simulink library "Lib_Piccolo"  (R2018b)
settings: Solver=VariableStepAuto  StartTime=0.0  StopTime=10.0  RelTol=1e-3
values from neighbouring files (symbols this model uses):
  AccelErrInt2Brakes = 0.15    [SimulationControlConfig16P.m]    (also in SimulationControlConfig16P_F0.m; SimulationControlConfig16P_F2.m; SimulationControlConfig16P_LEGACY.m; SimulationControlConfigTAILLESS.m = 0.2)
  AileronMax = 25    [SimulationControlConfig16P.m]    (also in SimulationControlConfig16P_F0.m; SimulationControlConfig16P_F2.m; SimulationControlConfig16P_LEGACY.m; SimulationControlConfigTAILLESS.m)
  AileronPower = 0.00268    [SimulationControlConfig16P.m]    (also in SimulationControlConfig16P_F0.m; SimulationControlConfig16P_F2.m; SimulationControlConfig16P_LEGACY.m; SimulationControlConfigTAILLESS.m = 0.002266)
  AileronSurfaceMax = 45    [SimulationControlConfig16P.m]    (also in SimulationControlConfig16P_F0.m; SimulationControlConfig16P_F2.m; SimulationControlConfig16P_LEGACY.m; SimulationControlConfigTAILLESS_CGAFT_F0.m = 25)
  AileronTrim = 0    [SimulationControlConfig16P.m]    (also in SimulationControlConfig16P_F0.m; SimulationControlConfig16P_F2.m; SimulationControlConfig16P_LEGACY.m; SimulationControlConfigTAILLESS.m)
  Alt = 1000 + TerrainHeight    [SimulationStateConfig.m]
  AltCruise_m = Alt * 0.3048    [SimulationControlConfig16P.m]    (also in SimulationControlConfig16P_F2.m; SimulationControlConfigTAILLESS.m = Alt/3.28084; SimulationControlConfigTAILLESS_CGAFT_F0.m = 640; SimulationControlConfigTAILLESS_CGFWD_F0.m = 640)
  AltitudeRate2PitchCmdIntegratorInit = 0.1    [SimulationControlPre.m]
  AltMax = 10000    [SimulationControlConfig16P.m]    (also in SimulationControlConfig16P_F0.m; SimulationControlConfig16P_F2.m; SimulationControlConfig16P_LEGACY.m; SimulationControlConfigTAILLESS.m)
  AltMaxAccel = 2.5    [SimulationControlConfig16P.m]    (also in SimulationControlConfig16P_F0.m = 2; SimulationControlConfig16P_F2.m = 2; SimulationControlConfig16P_LEGACY.m = 0.9; SimulationControlConfigTAILLESS.m = 2)
  AltMin = 0    [SimulationControlConfig16P.m]    (also in SimulationControlConfig16P_F0.m; SimulationControlConfig16P_F2.m; SimulationControlConfig16P_LEGACY.m; SimulationControlConfigTAILLESS.m)
  AltRateCmd2Pitch = 0.26    [SimulationControlConfig16P.m]    (also in SimulationControlConfig16P_F0.m = 0.35; SimulationControlConfig16P_F2.m = 0.35; SimulationControlConfig16P_LEGACY.m = 0.6; SimulationControlConfigTAILLESS.m = 0.9)
  AltRateError2Pitch = 0.34    [SimulationControlConfig16P.m]    (also in SimulationControlConfig16P_F0.m = 0.61; SimulationControlConfig16P_F2.m = 0.61; SimulationControlConfig16P_LEGACY.m = 0.4; SimulationControlConfigTAILLESS.m = 0.3)
  AltRateErrorInt2Pitch = 0.61    [SimulationControlConfig16P.m]    (also in SimulationControlConfig16P_F0.m = 0.28; SimulationControlConfig16P_F2.m = 0.28; SimulationControlConfig16P_LEGACY.m = 0.45; SimulationControlConfigTAILLESS.m = 0.15)
  AltRateLpfCutOff = 3    [SimulationControlConfig16P.m]    (also in SimulationControlConfig16P_F0.m; SimulationControlConfig16P_F2.m; SimulationControlConfig16P_LEGACY.m; SimulationControlConfigTAILLESS.m = 5)
  AutoNosegear2Rudder = 26    [SimulationControlConfig16P.m]    (also in SimulationControlConfig16P_F0.m; SimulationControlConfig16P_F2.m; SimulationControlConfig16P_LEGACY.m; SimulationControlConfigTAILLESS.m = 25.2)
  b = 5.54    [SimulationControlConfig16P.m]    (also in SimulationControlConfig16P_F0.m; SimulationControlConfig16P_F2.m; SimulationControlConfig16P_LEGACY.m; SimulationControlConfigTAILLESS.m = 2.37)
  Bank2AileronIntegratorInit = 0    [SimulationControlPre.m]
  BankMax_User = BankMax_User/180*pi    (= 0.610865238198)    [SimulationControlConfig16P.m]    (also in SimulationControlConfig16P_F0.m = 0.523598775598; SimulationControlConfig16P_F2.m = 0.523598775598; SimulationControlConfig16P_LEGACY.m = 0.523598775598; SimulationControlConfigTAILLESS.m = 0.558505360638)
  baseLegFlaps = 20    [SimulationControlConfig16P.m]    (also in SimulationControlConfig16P_F0.m; SimulationControlConfig16P_F2.m = 15; SimulationControlConfig16P_LEGACY.m = 0; SimulationControlConfigTAILLESS.m = 0)
  C = GeneticOpt.C    [SimulationCostFunction.m]
  c = Sw/b    (= 0.841696750903)    [SimulationControlConfig16P.m]    (also in SimulationControlConfig16P_F0.m; SimulationControlConfig16P_F2.m; SimulationControlConfig16P_LEGACY.m; SimulationControlConfigTAILLESS.m = 0.354008438819)
  cell2WheelFactorMG = 5.98    [SimulationSensorConfig16P_LEGACY.m]
  cell2WheelFactorNG = 1    [SimulationSensorConfig16P_LEGACY.m]
  cellSatMaxMG = 15000    [SimulationSensorConfig16P.m]    (also in SimulationSensorConfig16P_LEGACY.m; SimulationSensorConfigTAILLESS7P.m; SimulationSensorConfigUTAIL7P.m)
  cellSatMaxNG = 1000    [SimulationSensorConfig16P.m]    (also in SimulationSensorConfig16P_LEGACY.m; SimulationSensorConfigTAILLESS7P.m; SimulationSensorConfigUTAIL7P.m)
  cellSatMinMG = -15000    [SimulationSensorConfig16P.m]    (also in SimulationSensorConfig16P_LEGACY.m; SimulationSensorConfigTAILLESS7P.m; SimulationSensorConfigUTAIL7P.m)
  cellSatMinNG = -1000    [SimulationSensorConfig16P.m]    (also in SimulationSensorConfig16P_LEGACY.m; SimulationSensorConfigTAILLESS7P.m; SimulationSensorConfigUTAIL7P.m)
  CL_Limit = CL_Max    (= 0.54)    [SimulationControlConfig16P.m]    (also in SimulationControlConfig16P_F0.m; SimulationControlConfig16P_F2.m = 0.638; SimulationControlConfig16P_LEGACY.m; SimulationControlConfigTAILLESS.m = 0.525)
  CL_Max = 0.54    [SimulationControlConfig16P.m]    (also in SimulationControlConfig16P_F0.m; SimulationControlConfig16P_F2.m = 0.638; SimulationControlConfig16P_LEGACY.m; SimulationControlConfigTAILLESS.m = 0.525)
  CL_Max_Nom = 0.465    [SimulationControlConfig16P.m]    (also in SimulationControlConfig16P_F0.m; SimulationControlConfig16P_F2.m = 0.563; SimulationControlConfig16P_LEGACY.m; SimulationControlConfigTAILLESS.m = 0.39)
  CL_Min = 0    [SimulationControlConfig16P.m]    (also in SimulationControlConfig16P_F0.m; SimulationControlConfig16P_F2.m; SimulationControlConfig16P_LEGACY.m; SimulationControlConfigTAILLESS.m)
  ClimbMaxFraction = 0.35    [SimulationControlConfig16P.m]    (also in SimulationControlConfig16P_F0.m = 0.17; SimulationControlConfig16P_F2.m = 0.17; SimulationControlConfig16P_LEGACY.m = 0.24; SimulationControlConfigTAILLESS.m = 0.21)
  ClimboutMaxBank = 7.0    (= 7)    [SimulationControlConfig16P.m]    (also in SimulationControlConfig16P_F0.m; SimulationControlConfig16P_F2.m; SimulationControlConfig16P_LEGACY.m; SimulationControlConfigTAILLESS.m = 5)
  ClimboutTimer = 7.0    (= 7)    [SimulationControlConfig16P.m]    (also in SimulationControlConfig16P_F0.m; SimulationControlConfig16P_F2.m; SimulationControlConfig16P_LEGACY.m; SimulationControlConfigTAILLESS.m)
  dCl_per_dFlap = 0.005581818    [SimulationControlConfig16P.m]    (also in SimulationControlConfig16P_F0.m = 0; SimulationControlConfig16P_F2.m = 0.0065; SimulationControlConfig16P_LEGACY.m = 0; SimulationControlConfigTAILLESS.m = 0)
  DecelerationCmd = 3.1    [SimulationControlConfig16P.m]    (also in SimulationControlConfig16P_F0.m; SimulationControlConfig16P_F2.m; SimulationControlConfig16P_LEGACY.m; SimulationControlConfigTAILLESS.m = 0.1)
  DeRotateLogicEndTimer = abs((NoseDownLimit_Deg-1)/DeRotateRamp_Dps)    [SimulationControlConfig16P.m]    (also in SimulationControlConfig16P_F0.m; SimulationControlConfig16P_F2.m; SimulationControlConfig16P_LEGACY.m; SimulationControlConfigTAILLESS.m)
  DeRotateLogicHoldNoseUpTimer = 0.1    [SimulationControlConfig16P.m]    (also in SimulationControlConfig16P_F0.m; SimulationControlConfig16P_F2.m; SimulationControlConfig16P_LEGACY.m; SimulationControlConfigTAILLESS.m)
  DeRotateLogicTimerTimeout = 2    [SimulationControlConfig16P.m]    (also in SimulationControlConfig16P_F0.m; SimulationControlConfig16P_F2.m; SimulationControlConfig16P_LEGACY.m; SimulationControlConfigTAILLESS.m)
  DeRotateLowerCmdSaturation = 0    [SimulationControlConfig16P.m]    (also in SimulationControlConfig16P_F0.m; SimulationControlConfig16P_F2.m; SimulationControlConfig16P_LEGACY.m; SimulationControlConfigTAILLESS.m)
  DeRotateRamp_Dps = 3    [SimulationControlConfig16P.m]    (also in SimulationControlConfig16P_F0.m; SimulationControlConfig16P_F2.m; SimulationControlConfig16P_LEGACY.m; SimulationControlConfigTAILLESS.m = 8)
  DeRotateUpperCmdSaturation = 7    [SimulationControlConfig16P.m]    (also in SimulationControlConfig16P_F0.m; SimulationControlConfig16P_F2.m; SimulationControlConfig16P_LEGACY.m; SimulationControlConfigTAILLESS.m)
  DescentMaxFraction = 0.22    [SimulationControlConfig16P.m]    (also in SimulationControlConfig16P_F0.m = 0.2; SimulationControlConfig16P_F2.m = 0.2; SimulationControlConfig16P_LEGACY.m = 0.2; SimulationControlConfigTAILLESS.m = 0.17)
  DesktopSimTerrainOffset_m = 0.406    [SimulationAircraftConfig.m]
  downwindFlaps = 0    [SimulationControlConfig16P.m]    (also in SimulationControlConfig16P_F0.m; SimulationControlConfig16P_F2.m = 15; SimulationControlConfig16P_LEGACY.m; SimulationControlConfigTAILLESS.m)
  downwindSplitAil = 0    [SimulationControlConfig16P_F2.m]
  DP_init = 0.5*1.225*V_init^2    [SimulationControlConfig16P.m]    (also in SimulationControlConfig16P_F0.m; SimulationControlConfig16P_F2.m; SimulationControlConfig16P_LEGACY.m; SimulationControlConfigTAILLESS.m)
  dscNoiseMG = 1    [SimulationSensorConfig16P_LEGACY.m]
  dscNoiseNG = 0.25    [SimulationSensorConfig16P_LEGACY.m]
  DSCnumBits = 24    [SimulationSensorConfig16P.m]    (also in SimulationSensorConfig16P_LEGACY.m; SimulationSensorConfigTAILLESS7P.m; SimulationSensorConfigUTAIL7P.m)
  DSCRangeMaxMG = 15000    [SimulationSensorConfig16P.m]    (also in SimulationSensorConfig16P_LEGACY.m; SimulationSensorConfigTAILLESS7P.m; SimulationSensorConfigUTAIL7P.m)
  DSCRangeMaxNG = 1000    [SimulationSensorConfig16P.m]    (also in SimulationSensorConfig16P_LEGACY.m; SimulationSensorConfigTAILLESS7P.m; SimulationSensorConfigUTAIL7P.m)
  DSCRangeMinMG = -15000    [SimulationSensorConfig16P.m]    (also in SimulationSensorConfig16P_LEGACY.m; SimulationSensorConfigTAILLESS7P.m; SimulationSensorConfigUTAIL7P.m)
  DSCRangeMinNG = -1000    [SimulationSensorConfig16P.m]    (also in SimulationSensorConfig16P_LEGACY.m; SimulationSensorConfigTAILLESS7P.m; SimulationSensorConfigUTAIL7P.m)
  dt = DLLSim.dt    [SimulationTimeStep.m]    (also in SimulationTrim.m = 0.02)
  EarlyTouchdownThreshold = 3.0    (= 3)    [SimulationControlConfig16P.m]    (also in SimulationControlConfig16P_F0.m; SimulationControlConfig16P_F2.m; SimulationControlConfig16P_LEGACY.m; SimulationControlConfigTAILLESS.m)
  ElevatorDeflectionRate = 15    [SimulationControlConfig16P.m]    (also in SimulationControlConfig16P_F0.m; SimulationControlConfig16P_F2.m; SimulationControlConfig16P_LEGACY.m = 12; SimulationControlConfigTAILLESS.m = 5)
  ElevatorMax = 25    [SimulationControlConfig16P.m]    (also in SimulationControlConfig16P_F0.m; SimulationControlConfig16P_F2.m; SimulationControlConfig16P_LEGACY.m; SimulationControlConfigTAILLESS.m)
  ElevatorPower = -0.002209    [SimulationControlConfig16P.m]    (also in SimulationControlConfig16P_F0.m; SimulationControlConfig16P_F2.m; SimulationControlConfig16P_LEGACY.m; SimulationControlConfigTAILLESS.m = -0.002668)
  ElevatorTrim = -3.5    [SimulationControlConfig16P.m]    (also in SimulationControlConfig16P_F0.m; SimulationControlConfig16P_F2.m; SimulationControlConfig16P_LEGACY.m; SimulationControlConfigTAILLESS.m = -3)
  elevonBias = 0    [SimulationControlConfig16P.m]    (also in SimulationControlConfig16P_F0.m; SimulationControlConfig16P_F2.m; SimulationControlConfig16P_LEGACY.m; SimulationControlConfigTAILLESS.m)
  Enable_TAS_Protection = 0    [SimulationControlConfig16P.m]    (also in SimulationControlConfig16P_F0.m; SimulationControlConfig16P_F2.m; SimulationControlConfig16P_LEGACY.m; SimulationControlConfigTAILLESS.m)
  EnableCrossTrackAbort = 1    [SimulationControlConfig16P.m]    (also in SimulationControlConfigTAILLESS.m; SimulationControlConfigTAILLESS_CGAFT_F0.m; SimulationControlConfigTAILLESS_CGFWD_F0.m; SimulationControlConfigTAILLESS_CGFWD_F2.m)
  EnergyBandwidth = 0.04    [SimulationControlConfig16P.m]    (also in SimulationControlConfig16P_F0.m = 0.03; SimulationControlConfig16P_F2.m = 0.03; SimulationControlConfig16P_LEGACY.m = 0.02; SimulationControlConfigTAILLESS.m = 0.06)
  EngineLhFuelCut = 0    [SimulationAircraftConfig.m]
  EngineRhFuelCut = 0    [SimulationAircraftConfig.m]
  FastThrottleRate = 0.075    [SimulationControlConfig16P.m]    (also in SimulationControlConfig16P_F0.m = 0.05; SimulationControlConfig16P_F2.m = 0.05; SimulationControlConfig16P_LEGACY.m = 0.05; SimulationControlConfigTAILLESS.m = 0.1)
  FilterWarmUpTime = 2    [SimulationSensorConfig16P.m]    (also in SimulationSensorConfig16P_LEGACY.m; SimulationSensorConfigTAILLESS7P.m; SimulationSensorConfigUTAIL7P.m)
  finalApproachFlaps = 20    [SimulationControlConfig16P.m]    (also in SimulationControlConfig16P_F0.m; SimulationControlConfig16P_F2.m = 15; SimulationControlConfig16P_LEGACY.m = 0; SimulationControlConfigTAILLESS.m = 0)
  finalApproachSplitAil = 20    [SimulationControlConfig16P_F2.m]
  FinalDescentSlope_Deg = testPlans(testIndx).descentSlope    [SimulationControlConfig16P.m]    (also in SimulationControlConfig16P_F0.m; SimulationControlConfig16P_F2.m; SimulationControlConfig16P_LEGACY.m; SimulationControlConfigTAILLESS.m)
  flapMax = 0    [SimulationControlConfig16P.m]    (also in SimulationControlConfig16P_F0.m = 35; SimulationControlConfig16P_F2.m = 33; SimulationControlConfig16P_LEGACY.m; SimulationControlConfigTAILLESS.m)
  flapRate = 7.5    [SimulationControlConfig16P.m]    (also in SimulationControlConfig16P_F0.m; SimulationControlConfig16P_F2.m; SimulationControlConfig16P_LEGACY.m; SimulationControlConfigTAILLESS.m = 6.6)
  FlareHeight = 5    [SimulationControlConfig16P.m]    (also in SimulationControlConfig16P_F0.m; SimulationControlConfig16P_F2.m; SimulationControlConfig16P_LEGACY.m = 4.8; SimulationControlConfigTAILLESS.m = 2.75)
  FlareVerticalRate_mps = -0.4    [SimulationControlConfig16P.m]    (also in SimulationControlConfig16P_F0.m; SimulationControlConfig16P_F2.m; SimulationControlConfig16P_LEGACY.m = -0.5; SimulationControlConfigTAILLESS.m = -0.15)
  Fp_Aileron = 0.55*2*pi*RollRateLpfCutoff*dt    [SimulationControlConfig16P.m]    (also in SimulationControlConfig16P_F0.m; SimulationControlConfig16P_F2.m; SimulationControlConfig16P_LEGACY.m; SimulationControlConfigTAILLESS.m)
  Fp_Alt = 2*pi*0.55*AltBandwidth    (= 0.622035345411)    [SimulationControlConfig16P.m]    (also in SimulationControlConfig16P_F0.m; SimulationControlConfig16P_F2.m; SimulationControlConfig16P_LEGACY.m = 0.099; SimulationControlConfigTAILLESS.m = 0.207345115137)
  Fp_AltRate = 0.55*2*pi*AltRateLpfCutOff*dt    [SimulationControlConfig16P.m]    (also in SimulationControlConfig16P_F0.m; SimulationControlConfig16P_F2.m; SimulationControlConfig16P_LEGACY.m; SimulationControlConfigTAILLESS.m)
  Fp_Elevator = 0.55*2*pi*PitchRateLpfCutoff*dt    [SimulationControlConfig16P.m]    (also in SimulationControlConfig16P_F0.m; SimulationControlConfig16P_F2.m; SimulationControlConfig16P_LEGACY.m; SimulationControlConfigTAILLESS.m)
  Fp_Energy = 0.55*2*pi*EnergyBandwidth    (= 0.138230076758)    [SimulationControlConfig16P.m]    (also in SimulationControlConfig16P_F0.m = 0.103672557568; SimulationControlConfig16P_F2.m = 0.103672557568; SimulationControlConfig16P_LEGACY.m = 0.069115038379; SimulationControlConfigTAILLESS.m = 0.207345115137)
  Fp_Energy2 = 0.55*2*pi*EnergyBandwidth*dt    [SimulationControlConfig16P.m]    (also in SimulationControlConfig16P_F0.m; SimulationControlConfig16P_F2.m; SimulationControlConfig16P_LEGACY.m; SimulationControlConfigTAILLESS.m)
  Fp_Pitch = 0.55*2*pi*PitchBandwidth    (= 2.45358386245)    [SimulationControlConfig16P.m]    (also in SimulationControlConfig16P_F0.m; SimulationControlConfig16P_F2.m = 1.72787595947; SimulationControlConfig16P_LEGACY.m = 3.11017672705; SimulationControlConfigTAILLESS.m = 1.55508836353)
  Fp_Pitch_2 = 0.55*2*pi*PitchBandwidth*dt    [SimulationControlConfig16P.m]    (also in SimulationControlConfig16P_F0.m; SimulationControlConfig16P_F2.m; SimulationControlConfig16P_LEGACY.m; SimulationControlConfigTAILLESS.m)
  Fp_Roll = RollBandwidth^2    (= 1.69)    [SimulationControlConfig16P.m]    (also in SimulationControlConfig16P_F0.m = 1.44; SimulationControlConfig16P_F2.m = 1.44; SimulationControlConfig16P_LEGACY.m = 1.44; SimulationControlConfigTAILLESS.m = 1.21)
  Fp_Rudder = 0.55*2*pi*YawRateLpfCutoff*dt    [SimulationControlConfig16P.m]    (also in SimulationControlConfig16P_F0.m; SimulationControlConfig16P_F2.m; SimulationControlConfig16P_LEGACY.m; SimulationControlConfigTAILLESS.m)
  Fp_TAS = 0.55*2*pi*TASBandwidth    (= 0.103672557568)    [SimulationControlConfig16P.m]    (also in SimulationControlConfig16P_F0.m; SimulationControlConfig16P_F2.m; SimulationControlConfig16P_LEGACY.m; SimulationControlConfigTAILLESS.m = 0.172787595947)
  Fp_TAS_Filter = 2*pi*TasLpfCutoff*dt    [SimulationControlConfig16P.m]    (also in SimulationControlConfig16P_F0.m; SimulationControlConfig16P_F2.m; SimulationControlConfig16P_LEGACY.m; SimulationControlConfigTAILLESS.m)
  Fp_Turn = 0.55*2*pi*TurnErrLPFcutoff    (= 0.172787595947)    [SimulationControlConfig16P.m]    (also in SimulationControlConfig16P_F0.m = 0.0345575191895; SimulationControlConfig16P_F2.m = 0.0345575191895; SimulationControlConfig16P_LEGACY.m = 0.0345575191895; SimulationControlConfigTAILLESS.m)
  Fp_TurnDerr = 0.55*2*pi*TurnDerivativeLPFcutoff    (= 0.172787595947)    [SimulationControlConfig16P.m]    (also in SimulationControlConfig16P_F0.m = 0.0345575191895; SimulationControlConfig16P_F2.m = 0.0345575191895; SimulationControlConfig16P_LEGACY.m = 0.0345575191895; SimulationControlConfigTAILLESS.m)
  FTV = 3    [SimulationAircraftConfig.m]
  ftvStaticPositionError = 1/1.18    (= 0.847457627119)    [SimulationSensorConfig16P.m]    (also in SimulationSensorConfig16P_LEGACY.m; SimulationSensorConfigTAILLESS7P.m = 1; SimulationSensorConfigUTAIL7P.m = 1)
  g = 9.81    [SimulationStateConfig.m]
  goAroundSplitAil = 0    [SimulationControlConfig16P_F2.m]
  GustSpd_Kts = testPlans(testIndx).gustSpd    [SimulationStateConfig.m]
  GustTriggerVal = testPlans(testIndx).gustTriggerVal    [SimulationStateConfig.m]
  HeadingErr2TurnRate = 0.5    [SimulationControlConfig16P.m]    (also in SimulationControlConfig16P_F0.m; SimulationControlConfig16P_F2.m; SimulationControlConfig16P_LEGACY.m; SimulationControlConfigTAILLESS.m)
  HeadingErrDer2TurnRate = 0.3    [SimulationControlConfig16P.m]    (also in SimulationControlConfig16P_F0.m; SimulationControlConfig16P_F2.m; SimulationControlConfig16P_LEGACY.m; SimulationControlConfigTAILLESS.m)
  IASbounce = IASstall*0.8    [SimulationControlPre.m]
  IAScruiseCMD = sqrt(2*m*9.81/(1.225*Sw*CL_cruise))    [SimulationControlConfig16P.m]    (also in SimulationControlConfig16P_F0.m; SimulationControlConfig16P_F2.m; SimulationControlConfig16P_LEGACY.m; SimulationControlConfigTAILLESS.m)
  IASfinalCMD = 1.12 * IASmin    [SimulationControlConfig16P.m]    (also in SimulationControlConfig16P_F0.m = 1.14 * IASmin; SimulationControlConfig16P_F2.m = 1.10 * IASmin; SimulationControlConfig16P_LEGACY.m = 1.10 * IASmin; SimulationControlConfigTAILLESS.m = 1.14 * IASmin)
  IASflareCMD = IASstall    [SimulationControlConfig16P.m]    (also in SimulationControlConfig16P_F0.m; SimulationControlConfig16P_F2.m; SimulationControlConfig16P_LEGACY.m; SimulationControlConfigTAILLESS.m)
  IASmax = 64    [SimulationControlConfig16P.m]    (also in SimulationControlConfig16P_F0.m = 46; SimulationControlConfig16P_F2.m = 52; SimulationControlConfig16P_LEGACY.m = 46; SimulationControlConfigTAILLESS.m = 38.9)
  IASmin = sqrt(2*m*9.81/(1.225*Sw*0.9*CL_Max_Nom))    [SimulationControlConfig16P.m]    (also in SimulationControlConfig16P_F0.m; SimulationControlConfig16P_F2.m; SimulationControlConfig16P_LEGACY.m; SimulationControlConfigTAILLESS.m)
  IASshortCMD = IASstall    [SimulationControlConfig16P.m]    (also in SimulationControlConfig16P_F0.m; SimulationControlConfig16P_F2.m; SimulationControlConfig16P_LEGACY.m; SimulationControlConfigTAILLESS.m)
  IASstall = sqrt(2*m*9.81/(1.225*Sw*CL_Max))    [SimulationControlConfig16P.m]    (also in SimulationControlConfig16P_F0.m; SimulationControlConfig16P_F2.m; SimulationControlConfig16P_LEGACY.m; SimulationControlConfigTAILLESS.m)
  inFlight = 1    [SimulationControlConfig16P.m]    (also in SimulationControlConfigTAILLESS.m; SimulationControlConfigTAILLESS_CGAFT_F0.m; SimulationControlConfigTAILLESS_CGFWD_F0.m; SimulationControlConfigTAILLESS_CGFWD_F2.m)
  JetCatOffset = 5    [SimulationControlConfig16P.m]    (also in SimulationControlConfig16P_F0.m; SimulationControlConfig16P_F2.m; SimulationControlConfig16P_LEGACY.m)
  LaunchRollingElevator = -1.5    [SimulationControlConfig16P.m]    (also in SimulationControlConfig16P_F0.m; SimulationControlConfig16P_F2.m = 1.25; SimulationControlConfig16P_LEGACY.m; SimulationControlConfigTAILLESS.m = 1)
  ldg_NosegearMax = 10    [SimulationControlConfig16P.m]    (also in SimulationControlConfig16P_F0.m; SimulationControlConfig16P_F2.m; SimulationControlConfig16P_LEGACY.m; SimulationControlConfigTAILLESS.m)
  ldg_TrackVyErrInt2Nosegear = 0.1250    (= 0.125)    [SimulationControlConfig16P.m]    (also in SimulationControlConfig16P_F0.m; SimulationControlConfig16P_F2.m; SimulationControlConfig16P_LEGACY.m; SimulationControlConfigTAILLESS.m = 0.00714285714286)
  ldg_TrackVyErrPro2Nosegear = 0.35    [SimulationControlConfig16P.m]    (also in SimulationControlConfig16P_F0.m; SimulationControlConfig16P_F2.m; SimulationControlConfig16P_LEGACY.m; SimulationControlConfigTAILLESS.m = 0.0546666666667)
  ldg_TrackY2Vy = 0.07    [SimulationControlConfig16P.m]    (also in SimulationControlConfig16P_F0.m; SimulationControlConfig16P_F2.m; SimulationControlConfig16P_LEGACY.m; SimulationControlConfigTAILLESS.m = 0.17)
  ldg_Vy2NosegearScalingPower = 1.075    [SimulationControlConfig16P.m]    (also in SimulationControlConfig16P_F0.m; SimulationControlConfig16P_F2.m; SimulationControlConfig16P_LEGACY.m; SimulationControlConfigTAILLESS.m = 0.6)
  ldg_Y2VyScalingPower = 0.175    [SimulationControlConfig16P.m]    (also in SimulationControlConfig16P_F0.m; SimulationControlConfig16P_F2.m; SimulationControlConfig16P_LEGACY.m; SimulationControlConfigTAILLESS.m = 0)
  ldg_YawRate2Nosegear = 0.175    [SimulationControlConfig16P.m]    (also in SimulationControlConfig16P_F0.m; SimulationControlConfig16P_F2.m; SimulationControlConfig16P_LEGACY.m; SimulationControlConfigTAILLESS.m = 0.065)
  LiftSlope = 0.064285    [SimulationControlConfig16P.m]    (also in SimulationControlConfig16P_F0.m; SimulationControlConfig16P_F2.m; SimulationControlConfig16P_LEGACY.m; SimulationControlConfigTAILLESS.m = 0.058631)
  LPFaileronInit = 0    [SimulationControlPre.m]
  LPFclestInit = 0    [SimulationControlPre.m]
  LPFenergyFFInit = 0    [SimulationControlPre.m]
  ... (+122 more)
undefined symbols (not defined in the file or in its folder): abortFlag, alphaHPF, apmDelay, BRWNOUT, CRAWOR, CRAWUR, DiscIntNeverNeededParam, DLLSim, DLLSimStep, ECOMOR, ECOMUR, Fp_Tas, GustTrigger_HeightAgl_m, IPSTAT, LCINTEG, Ldg_Persist_Time, LOWER_FLAGS, MSG_ENABLE, NoiseStd, OLDVAL, OVERRIDE_ENABLE, OVERRIDE_VALUE, REBOOT, reversionEnable, revIASMax, revIASMin, revPitchMax, revPitchMin, revPitchRateMax, revRollMax, revRollRateMax, SAMPLE, SCALON, SensorModel, sigbuilder_block, Sim_Vx, Sim_Vy, Sim_Vz, Sim_Xpos, Sim_Ypos, Sim_Zpos, SYSOR, SYSUR, TARE, TEMPOR, TEMPUR, testIndx, testPlan, testPlans, Trim_piccoloInCmd, Trim_REFSI_FD_IN_nmodeCgShifterCmd_Flag, Trim_REFSI_FD_IN_nmodeCgShifterCmd_Ft, Trim_REFSI_FD_IN_nmodeCgShifterCmdType, Trim_REFSI_FD_IN_nmodeCgShifterNRCActive, Trim_REFSI_FD_IN_nmodeFlapLhIBCmd_Deg, Trim_REFSI_FD_IN_nmodeFlapLhOBCmd_Deg, Trim_REFSI_FD_IN_nmodeFlapRhIBCmd_Deg, Trim_REFSI_FD_IN_nmodeFlapRhOBCmd_Deg, Trim_REFSI_FD_IN_nmodeSlatLhCmd_Deg ... (+11)
libraries: simulink x1237, $bdroot x179, aerolibconvert2 x63, dspswit3 x25, aerolibatmos2 x5, simulink_extras x4, dsparch4 x2, Lib_Piccolo_Alt x2, eeGeneralControl x1, dspindex x1
(part 10 of 74)

== system Lib_Piccolo/Bank to Aileron/Bank Angle Limit Calculation ==
  note: From FWG3 Doc (Page 13) -
      | if (state >= shortFinal)
      | $C_{L-Limit} =C_{L-MAX}$
      | else
      | $C_{L-Limit} = 0.9C_{L-MAX\_NOM}$
      |
      | Adjustments will need to be applied to CL_Limit here,
      | CL_Limit = CL_Limit + dCl/dFlap * dFlap
  note: Leave Aero Load Feature off During Landing Verification
      | (switch in down position)
  apMode : Inport
  Q : Inport  Port=2
  Acos : Trigonometry  Operator=acos
  Compare To Constant1 : simulink/Logic and Bit Operations/Compare To Constant  relop=<=  const=9  OutDataTypeStr=uint8
  Compare To Constant2 : simulink/Logic and Bit Operations/Compare To Constant  relop=>=  const=9  OutDataTypeStr=uint8
  Constant : Constant  Value=Sw
  Constant1 : Constant  Value=CL_Limit
  Constant2 : Constant  Value=m
  Constant3 : Constant  Value=nMax_User
  Constant4 : Constant  Value=nMin_User
  Constant5 : Constant  Value=CL_Min
  Constant6 : Constant
  Constant7 : Constant  Value=0.9*CL_Max_Nom
  Divide : Product  Inputs=*/
  Flap Compensation : $bdroot/Pitch to Elevator/Reference Frame Conversion and Pitch Rate Limit Determination/AeroVsStruct_Limit/Flap Compensation  SystemSampleTime=-1
  Gain9 : Gain  Gain=180/pi
  "Load Factors (nMax,nMin) at current conditions " : MATLAB Function  TreatAsAtomicUnit=on
  Min : MinMax  Inputs=2
  Switch : Switch  Criteria=u2 > Threshold
  Switch1 : Switch  Criteria=u2 > Threshold
  Terminator : Terminator
  Terminator2 : Terminator
  "User and State Machine Limits " : Subsystem
  BankMax_Euler : Outport
  wires:
  Flap Compensation/1 -> "Load Factors (nMax,nMin) at current conditions "/3(CL_Limit)  "Sim.CL_Limit"
  Constant7/1 -> Switch1/3
  Switch1/1 -> Flap Compensation/1
  Constant1/1 -> Switch1/1
  Compare To Constant2/1 -> Switch1/2
  apMode/1 -> "User and State Machine Limits "/1(apMode), Compare To Constant1/1, Compare To Constant2/1
  Switch/1 -> BankMax_Euler/1
  Compare To Constant1/1 -> Switch/2
  "User and State Machine Limits "/1(UserLimit) -> Switch/3, Min/2
  Gain9/1 -> Terminator2/1  "Sim.BanknMax"
  Acos/1 -> Min/1, Gain9/1
  Min/1 -> Switch/1
  Divide/1 -> Acos/1
  Constant6/1 -> Divide/1
  "Load Factors (nMax,nMin) at current conditions "/2(nMin) -> Terminator/1
  Constant5/1 -> "Load Factors (nMax,nMin) at current conditions "/4(CL_Min)
  Constant4/1 -> "Load Factors (nMax,nMin) at current conditions "/7(nMin_User)
  Constant3/1 -> "Load Factors (nMax,nMin) at current conditions "/6(nMax_User)
  Constant2/1 -> "Load Factors (nMax,nMin) at current conditions "/5(m)
  Constant/1 -> "Load Factors (nMax,nMin) at current conditions "/2(Sw)
  "Load Factors (nMax,nMin) at current conditions "/1(nMax) -> Divide/2  "nMax"
  Q/1 -> "Load Factors (nMax,nMin) at current conditions "/1(Q)

== system Lib_Piccolo/Bank to Aileron/Dynamic Inversion PID ==
  RollRateCmd_Euler : Inport
  RollRate_Euler : Inport  Port=2
  Q : Inport  Port=3
  V : Inport  Port=4
  apMode : Inport  Port=5
  1-K_TD : Gain  Gain=1-RollDampingTrust
  1/AileronPower : Gain  Gain=1/AileronPower
  "1/AileronPower  " : Gain  Gain=1/AileronPower
  "AileronTrim " : Constant  Value=AileronTrim
  Compare To Constant1 : simulink/Logic and Bit Operations/Compare To Constant  relop=<=  const=1  OutDataTypeStr=uint8
  Compare To Constant2 : simulink/Logic and Bit Operations/Compare To Constant  relop===  const=11  OutDataTypeStr=uint8
  Constant2 : Constant  Value=Bank2AileronIntegratorInit
  Dimensional Aileron Power : Subsystem
  Discrete-Time Integrator1 : DiscreteIntegrator  IntegratorMethod=Integration: Backward Euler  gainval=1  ExternalReset=level  InitialConditionSource=external  SampleTime=-1  LimitOutput=on  UpperSaturationLimit=AileronMax  LowerSaturationLimit=-AileronMax  ICPrevOutput=DiscIntNeverNeededParam  ICPrevScaledInput=DiscIntNeverNeededParam
  Divide : Product  Inputs=/*
  Gain : Gain  Gain=-1
  Gain1 : Gain
  Gain4 : Gain  Gain=RollRateError2Accel
  KI_Roll : Gain  Gain=RollRateErrorInt2Accel
  K_TD : Gain  Gain=RollDampingTrust
  Kp_Roll : Gain  Gain=RollRateError2Accel
  LPF AileronCmd : Subsystem
  NOT : Logic  Operator=NOT  IconShape=distinctive  AllPortsSameDT=off  OutDataTypeStr=boolean
  NOT1 : Logic  Operator=NOT  IconShape=distinctive  AllPortsSameDT=off  OutDataTypeStr=boolean
  OR : Logic  Operator=OR  IconShape=distinctive  AllPortsSameDT=off  OutDataTypeStr=boolean
  OR1 : Logic  Operator=OR  IconShape=distinctive  AllPortsSameDT=off  OutDataTypeStr=boolean
  Roll Moment Caused By Damping : Subsystem
  Rollout Roll Control : Subsystem
  STIFF : Constant  Value=0
  Saturation : Saturate  UpperLimit=AileronMax  LowerLimit=-AileronMax
  Saturation1 : Saturate  UpperLimit=6125  LowerLimit=200
  Sum : Sum  Inputs=|+-
  Sum1 : Sum  Inputs=|+--+
  Sum2 : Sum  Inputs=|++
  Sum3 : Sum  Inputs=++|
  Switch : Switch  Criteria=u2 > Threshold
  Terminator : Terminator
  Terminator1 : Terminator
  Unit Delay : UnitDelay  SampleTime=-1
  Aileron_Deg : Outport
  wires:
  Saturation1/1 -> Dimensional Aileron Power/1(Dynamic Pressure (Avoid Small Value))
  NOT/1 -> Switch/2
  Rollout Roll Control/1(Aileron Out) -> Saturation/1
  LPF AileronCmd/1(Output) -> Rollout Roll Control/2(Aileron In)
  Compare To Constant2/1 -> OR/1
  apMode/1 -> Compare To Constant2/1, Compare To Constant1/1, Rollout Roll Control/1(apMode)
  Compare To Constant1/1 -> OR/2
  OR1/1 -> Discrete-Time Integrator1/2, Unit Delay/1
  1/AileronPower/1 -> Gain/1, Sum1/2
  Roll Moment Caused By Damping/1(DAMP) -> 1/AileronPower/1
  Discrete-Time Integrator1/1 -> Sum3/1  "Sim_KI_roll"
  Kp_Roll/1 -> Sum3/2  "Sim_Kp_roll"
  Sum3/1 -> Switch/1
  Constant2/1 -> Discrete-Time Integrator1/3
  KI_Roll/1 -> Discrete-Time Integrator1/1
  Dimensional Aileron Power/1(CP) -> Divide/1
  Sum/1 -> Divide/2  "Sim.RollRate Error"
  Gain4/1 -> Switch/3  "Sim_Kp_roll"
  RollRate_Euler/1 -> Sum/2, K_TD/1
  RollRateCmd_Euler/1 -> 1-K_TD/1, Sum/1
  Unit Delay/1 -> NOT/1
  Switch/1 -> Gain1/1
  Gain1/1 -> Sum1/1
  Gain/1 -> Terminator/1  "Sim_RollDamping"
  Saturation/1 -> Aileron_Deg/1
  1-K_TD/1 -> Sum2/1
  Divide/1 -> Gain4/1, Kp_Roll/1, KI_Roll/1
  Sum2/1 -> Roll Moment Caused By Damping/1(RollRate_Body)  "RollDamp_TrustMix"
  V/1 -> Roll Moment Caused By Damping/2(V)
  "AileronTrim "/1 -> Sum1/4
  "1/AileronPower  "/1 -> Sum1/3
  K_TD/1 -> Sum2/2
  STIFF/1 -> "1/AileronPower  "/1
  Sum1/1 -> LPF AileronCmd/1("Input ")
  Q/1 -> Saturation1/1
  [ApGlobal] -> NOT1/1
  OR/1 -> OR1/1
  NOT1/1 -> Terminator1/1, OR1/2

== system Lib_Piccolo/Bank to Aileron/DynamicPLimit ==
  note: Q saturates at ~ 100mps which in IAS is 6125Pa
  apMode : Inport
  DynamicPressure_Pa : Inport  Port=2
  Compare To Constant1 : simulink/Logic and Bit Operations/Compare To Constant  relop=>=  const=5  OutDataTypeStr=uint8
  Compare To Constant2 : simulink/Logic and Bit Operations/Compare To Constant  relop=>=  const=11  OutDataTypeStr=uint8
  Compare To Constant3 : simulink/Logic and Bit Operations/Compare To Constant  relop=>=  const=10  OutDataTypeStr=uint8
  Latch : Subsystem
  Qmax : Constant  Value=6125
  Saturation Dynamic : simulink/Discontinuities/Saturation Dynamic  OutMin=[]  OutMax=[]  OutDataTypeStr=Inherit: Same as second input  OutDataType=fixdt(1, 16)  OutScaling=2^-10  DoSatur=off
  Switch : Switch  Criteria=u2 > Threshold
  Switch1 : Switch  Criteria=u2 > Threshold
  Out1 : Outport
  wires:
  Latch/1(Q_Latched) -> Switch1/2
  Switch1/1 -> Saturation Dynamic/3
  [Qmin_Bounce] -> Switch1/1
  Switch/1 -> Switch1/3
  Compare To Constant2/1 -> Latch/1(D)
  Compare To Constant1/1 -> Latch/2(Enable/!Rst)
  Qmax/1 -> Saturation Dynamic/1
  [Qmin_Flare] -> Switch/1
  [Qmin] -> Switch/3
  Compare To Constant3/1 -> Switch/2
  apMode/1 -> Compare To Constant3/1, Compare To Constant2/1, Compare To Constant1/1
  Saturation Dynamic/1 -> Out1/1
  DynamicPressure_Pa/1 -> Saturation Dynamic/2

== system Lib_Piccolo/Bank to Aileron/Reference Model ==
  BankCmd_Euler : Inport
  "Bank_Euler " : Inport  Port=2
  "BankMax_Euler " : Inport  Port=3
  Constant : Constant  Value=RollMaxAccel
  Fp_roll : Gain  Gain=Fp_Roll
  Gain1 : Gain  Gain=-1
  Gain2 : Gain  Gain=-1
  Gain3 : Gain  Gain=-1
  Gain4 : Gain  Gain=180/pi
  Gain9 : Gain  Gain=180/pi
  Roll Rate Max Accel Rate Limit : Subsystem
  "RollRateCmd " : Constant  Value=0
  "RollRateLimit_Max " : Constant  Value=RollRateMax
  Saturation Dynamic : simulink/Discontinuities/Saturation Dynamic  OutMin=[]  OutMax=[]  OutDataTypeStr=Inherit: Same as second input  OutDataType=fixdt(1, 16)  OutScaling=2^-10  DoSatur=off
  Saturation Dynamic1 : simulink/Discontinuities/Saturation Dynamic  OutMin=[]  OutMax=[]  OutDataTypeStr=Inherit: Same as second input  OutDataType=fixdt(1, 16)  OutScaling=2^-10  DoSatur=off
  Sum : Sum  Inputs=|+-
  Sum1 : Sum  Inputs=|++
  Terminator : Terminator
  Terminator2 : Terminator
  RollRateCmd_Euler : Outport
  tag scope: Sim_BankCmd=global
  wires:
  Saturation Dynamic1/1 -> Sum/1, Gain4/1, [Sim_BankCmd]
  Saturation Dynamic/1 -> RollRateCmd_Euler/1
  Gain9/1 -> Terminator2/1  "Sim.BankLimit"
  BankCmd_Euler/1 -> Saturation Dynamic1/2
  "RollRateLimit_Max "/1 -> Gain3/1, Saturation Dynamic/1
  Constant/1 -> Gain1/1, Roll Rate Max Accel Rate Limit/1(up)
  Fp_roll/1 -> Sum1/1
  Gain2/1 -> Saturation Dynamic1/3
  Gain4/1 -> Terminator/1  "Sim.BankCmd_Limit"
  Roll Rate Max Accel Rate Limit/1(Y) -> Saturation Dynamic/2
  Sum1/1 -> Roll Rate Max Accel Rate Limit/2(u)
  Gain3/1 -> Saturation Dynamic/3
  "BankMax_Euler "/1 -> Gain2/1, Saturation Dynamic1/1, Gain9/1
  Sum/1 -> Fp_roll/1
  "Bank_Euler "/1 -> Sum/2
  Gain1/1 -> Roll Rate Max Accel Rate Limit/3(lo)
  "RollRateCmd "/1 -> Sum1/2

== system Lib_Piccolo/Bank to Aileron/TASLimit ==
  note: TAS saturates at ~ 100mps which in IAS is 6125Pa
  apMode : Inport
  <V_mps> : Inport  Port=2
  Compare To Constant1 : simulink/Logic and Bit Operations/Compare To Constant  relop=>=  const=5  OutDataTypeStr=uint8
  Compare To Constant2 : simulink/Logic and Bit Operations/Compare To Constant  relop=>=  const=11  OutDataTypeStr=uint8
  Compare To Constant4 : simulink/Logic and Bit Operations/Compare To Constant  relop=>=  const=10  OutDataTypeStr=uint8
  Constant : Constant  Value=IASmin
  Constant1 : Constant  Value=IASstall
  Constant2 : Constant  Value=IASbounce
  Latch : Subsystem
  Saturation Dynamic1 : simulink/Discontinuities/Saturation Dynamic  OutMin=[]  OutMax=[]  OutDataTypeStr=Inherit: Same as second input  OutDataType=fixdt(1, 16)  OutScaling=2^-10  DoSatur=off
  Switch1 : Switch  Criteria=u2 > Threshold
  Switch2 : Switch  Criteria=u2 > Threshold
  TASmax : Constant  Value=100
  Out1 : Outport
  wires:
  TASmax/1 -> Saturation Dynamic1/1
  Constant2/1 -> Switch2/1
  Compare To Constant1/1 -> Latch/2(Enable/!Rst)
  Switch1/1 -> Switch2/3
  apMode/1 -> Compare To Constant4/1, Compare To Constant2/1, Compare To Constant1/1
  Compare To Constant2/1 -> Latch/1(D)
  Latch/1(Q_Latched) -> Switch2/2
  <V_mps>/1 -> Saturation Dynamic1/2
  Constant/1 -> Switch1/3
  Saturation Dynamic1/1 -> Out1/1
  Constant1/1 -> Switch1/1
  Compare To Constant4/1 -> Switch1/2
  Switch2/1 -> Saturation Dynamic1/3

== system Lib_Piccolo/Brake Controller/Variant Subsystem ==
  note: 1) Add Subsystem or Model blocks as valid variant choices.
      | 2) You cannot connect blocks at this level. At simulation, connectivity is automatically
      | determined, based on the active variant and port name matching.
  Feedback Bus : Inport
  16P : Subsystem  VariantControl="modelScale ==\"16P5\""
  7P : Subsystem  VariantControl="modelScale == \"7P\""
  Brake_Pcnt : Outport

== system Lib_Piccolo/Control Allocation/M2 ==
  note: For 16.5% U-tail:
      | Aileron: aileron, inboard elevon, outboard elevon
      | Elevator: aft-flap, U-tail elevator,
      | Rudder: pylon rudder, winglet rudder, U-tail rudder
      |
      | For 16.5% Tailless (w/o U-tail elevator and U-tail rudder):
      | Aileron: aileron, inboard elevon, outboard elevon
      | Elevator: aft-flap, inboard elvon, outboard elevon
      | Rudder: pylon rudder, winglet rudder
  Aileron : Inport
  Elevator : Inport  Port=2
  Rudder : Inport  Port=3
  Throttle : Inport  Port=4
  Nosegear : Inport  Port=5
  Brake : Inport  Port=6
  Flap : Inport  Port=7
  HStab : Inport  Port=8
  Feedback Bus : Inport  Port=9
  Bus Creator : BusCreator  Inputs=10
  Bus Creator1 : BusCreator  Inputs=4
  Bus Creator2 : BusCreator  Inputs=2
  Bus Creator3 : BusCreator  Inputs=2
  Bus Creator4 : BusCreator  Inputs=2
  Constant : Constant  Value=FTV
  Constant1 : Constant  Value=0
  Constant2 : Constant  Value=elevonBias
  Gain{1..5,8..9,12,14,16..17} (11 alike) : Gain
  Gain{10..11,13,15} (4 alike) : Gain  Gain=-1
  Signal Specification : SignalSpecification  Dimensions=[1 1]  SampleTime=dt
  Signal Specification1 : SignalSpecification  Dimensions=[1 1]  SampleTime=dt
  Signal Specification2 : SignalSpecification  Dimensions=[1 1]  SampleTime=dt
  SlatLhPosnDeg : Constant  Value=Trim_REFSI_FD_IN_nmodeSlatLhCmd_Deg
  Surface Mixing Function : MATLAB Function  TreatAsAtomicUnit=on
  Switch : Switch  Criteria=u2 > Threshold  Threshold=2
  Terminator : Terminator
  Variant Model : $bdroot/Control Allocation/M2 Flap-to-Drag /Variant Model  SystemSampleTime=-1
  nmodeTlaLhCmdDeg3 : Constant  Value=Trim_REFSI_FD_IN_nmodeSplrLhOutbdCmd_Deg
  "Aileron_Deg " : Outport
  "InboardElevon_Deg " : Outport  Port=2
  OutboardElevon_Deg : Outport  Port=3
  "U-TailElevator_Deg " : Outport  Port=4
  Aft-Flap_Deg : Outport  Port=5
  PylonRudder_Deg : Outport  Port=6
  WingletRudder_Deg : Outport  Port=7
  U-tailRudder_Deg : Outport  Port=8
  "Throttle_Pct " : Outport  Port=9
  Nosegear_Deg : Outport  Port=10
  Brake (0-1) : Outport  Port=11
  Flaps_Deg : Outport  Port=12
  Slats_Deg : Outport  Port=13
  Spoilers_Deg : Outport  Port=14
  Stabilizer_Deg : Outport  Port=15
  tag scope: Sim_Surface=global
  wires:
  Elevator/1 -> Bus Creator/2, Signal Specification1/1  "Sim_ElevatorCmd"
  Aileron/1 -> Bus Creator/1, Signal Specification/1  "Sim_AileronCmd"
  Rudder/1 -> Bus Creator/3, Signal Specification2/1  "Sim_RudderCmd"
  Nosegear/1 -> Bus Creator/5, Nosegear_Deg/1  "Sim_NosegearCmd"
  Brake/1 -> Brake (0-1)/1, Bus Creator/6  "Sim_BrakeCmd"
  Bus Creator/1 -> [Sim_Surface]
  Throttle/1 -> Variant Model/1, Bus Creator/4  "Sim_ThrottleCmd"
  Variant Model/1 -> Gain16/1, Gain17/1  "Sim_ThrottleCmd"
  Bus Creator1/1 -> "Aileron_Deg "/1
  Bus Creator2/1 -> "InboardElevon_Deg "/1
  Bus Creator3/1 -> OutboardElevon_Deg/1
  Gain8/1 -> Bus Creator1/1  "PrtAileronUpperCmd_Deg"
  Gain9/1 -> Bus Creator1/2  "PrtAileronLowerCmd_Deg"
  Gain10/1 -> Bus Creator1/3  "StbdAileronUpperCmd_Deg"
  Gain11/1 -> Bus Creator1/4  "StbdAileronLowerCmd_Deg"
  Gain12/1 -> Bus Creator2/1  "PrtInbElevonCmd_Deg"
  Gain13/1 -> Bus Creator2/2  "StbdInbElevonCmd_Deg"
  Gain14/1 -> Bus Creator3/1  "PrtOutElevonCmd_Deg"
  Gain15/1 -> Bus Creator3/2  "StbdOutElevonCmd_Deg"
  Gain16/1 -> Bus Creator4/1  "PrtThrottleCmd_Pct"
  Bus Creator4/1 -> "Throttle_Pct "/1
  Gain17/1 -> Bus Creator4/2  "StbdThrottleCmd_Pct"
  SlatLhPosnDeg/1 -> Bus Creator/8, Slats_Deg/1  "Sim_SlatsCmd"
  nmodeTlaLhCmdDeg3/1 -> Bus Creator/9, Spoilers_Deg/1  "Sim_SpoilersCmd"
  Feedback Bus/1 -> Terminator/1
  HStab/1 -> Bus Creator/10, Stabilizer_Deg/1  "Sim_StabilizerCmd"
  Flap/1 -> Surface Mixing Function/4(Pic_FlapCmd), Bus Creator/7, Flaps_Deg/1  "Sim_FlapCmd"
  Surface Mixing Function/1(PrtAileronUpperCmd) -> Gain8/1
  Surface Mixing Function/2(PrtAileronLowerCmd) -> Gain9/1
  Surface Mixing Function/3(StbdAileronUpperCmd) -> Gain10/1
  Surface Mixing Function/4(StbdAileronLowerCmd) -> Gain11/1
  Surface Mixing Function/13(UTailRudderCmd) -> Gain5/1
  Surface Mixing Function/12(WingletRudderCmd) -> Gain4/1
  Surface Mixing Function/11(PylonRudderCmd) -> Gain3/1
  Surface Mixing Function/10(AftFlapCmd) -> Gain2/1
  Surface Mixing Function/9(ElevatorUtailCmd) -> Gain1/1
  Surface Mixing Function/8(StbdOutdElevonCmd) -> Gain15/1
  Surface Mixing Function/7(PrtOutElevonCmd) -> Gain14/1
  Surface Mixing Function/6(StbdInbdElevonCmd) -> Gain13/1
  Surface Mixing Function/5(PrtInbElevonCmd) -> Gain12/1
  Gain1/1 -> "U-TailElevator_Deg "/1  "UtailElevator_Deg"
  Gain2/1 -> Aft-Flap_Deg/1  "AftFlap_deg"
  Gain3/1 -> PylonRudder_Deg/1  "PylonRudder_Deg"
  Gain5/1 -> U-tailRudder_Deg/1  "UtailRudder_Deg"
  Signal Specification/1 -> Surface Mixing Function/1(Pic_AileronCmd)
  Signal Specification2/1 -> Surface Mixing Function/3(Pic_RudderCmd)
  Signal Specification1/1 -> Surface Mixing Function/2(Pic_ElevatorCmd)
  Constant/1 -> Switch/2
  Switch/1 -> WingletRudder_Deg/1  "WingletRudder_Deg"
  Constant1/1 -> Switch/3
  Gain4/1 -> Switch/1
  Constant2/1 -> Surface Mixing Function/5(elevonBias)

== system Lib_Piccolo/Control Allocation/M2 Built-In-SplitAil ==
  note: For 16.5% U-tail:
      | Aileron: aileron, inboard elevon, outboard elevon
      | Elevator: aft-flap, U-tail elevator,
      | Rudder: pylon rudder, winglet rudder, U-tail rudder
      |
      | For 16.5% Tailless (w/o U-tail elevator and U-tail rudder):
      | Aileron: aileron, inboard elevon, outboard elevon
      | Elevator: aft-flap, inboard elvon, outboard elevon
      | Rudder: pylon rudder, winglet rudder
  Aileron : Inport
  Elevator : Inport  Port=2
  Rudder : Inport  Port=3
  Throttle : Inport  Port=4
  Nosegear : Inport  Port=5
  Brake : Inport  Port=6
  Flap : Inport  Port=7
  HStab : Inport  Port=8
  Feedback Bus : Inport  Port=9
  Bus Creator : BusCreator  Inputs=11
  Bus Creator1 : BusCreator  Inputs=4
  Bus Creator2 : BusCreator  Inputs=2
  Bus Creator3 : BusCreator  Inputs=2
  Bus Creator4 : BusCreator  Inputs=2
  Constant : Constant  Value=FTV
  Constant1 : Constant  Value=0
  Constant2 : Constant  Value=elevonBias
  Constant3 : Constant  Value=AileronSurfaceMax
  FlapLhIBCmdDeg : Constant  Commented=on  Value=Trim_REFSI_FD_IN_nmodeFlapLhIBCmd_Deg
  Gain{1..5,8..9,12,14,16..17} (11 alike) : Gain
  Gain{10..11,13,15} (4 alike) : Gain  Gain=-1
  Signal Specification{,1..3} (4 alike) : SignalSpecification  Dimensions=[1 1]  SampleTime=dt
  SlatLhPosnDeg : Constant  Value=Trim_REFSI_FD_IN_nmodeSlatLhCmd_Deg
  Split Aileron Deployment : Subsystem
  Surface Mixing Function : MATLAB Function  TreatAsAtomicUnit=on
  Switch : Switch  Criteria=u2 > Threshold  Threshold=2
  Variant Model : Subsystem  Variant=on
  nmodeTlaLhCmdDeg3 : Constant  Value=Trim_REFSI_FD_IN_nmodeSplrLhOutbdCmd_Deg
  "Aileron_Deg " : Outport
  "InboardElevon_Deg " : Outport  Port=2
  OutboardElevon_Deg : Outport  Port=3
  "U-TailElevator_Deg " : Outport  Port=4
  Aft-Flap_Deg : Outport  Port=5
  PylonRudder_Deg : Outport  Port=6
  WingletRudder_Deg : Outport  Port=7
  U-tailRudder_Deg : Outport  Port=8
  "Throttle_Pct " : Outport  Port=9
  Nosegear_Deg : Outport  Port=10
  Brake (0-1) : Outport  Port=11
  Flaps_Deg : Outport  Port=12
  Slats_Deg : Outport  Port=13
  Spoilers_Deg : Outport  Port=14
  Stabilizer_Deg : Outport  Port=15
  tag scope: Sim_Surface=global
  wires:
  Split Aileron Deployment/1(SplitAileron_Cmd) -> Signal Specification3/1, Bus Creator/8  "Sim_SplitAileronCmd"
  Feedback Bus/1 -> Split Aileron Deployment/1(FeedbackBus)
  Gain4/1 -> Switch/1
  Constant1/1 -> Switch/3
  Switch/1 -> WingletRudder_Deg/1  "WingletRudder_Deg"
  Constant/1 -> Switch/2
  Signal Specification1/1 -> Surface Mixing Function/2(Pic_ElevatorCmd)
  Signal Specification2/1 -> Surface Mixing Function/3(Pic_RudderCmd)
  Signal Specification/1 -> Surface Mixing Function/1(Pic_AileronCmd)
  Gain5/1 -> U-tailRudder_Deg/1  "UtailRudder_Deg"
  Gain3/1 -> PylonRudder_Deg/1  "PylonRudder_Deg"
  Gain2/1 -> Aft-Flap_Deg/1  "AftFlap_deg"
  Gain1/1 -> "U-TailElevator_Deg "/1  "UtailElevator_Deg"
  Surface Mixing Function/5(PrtInbElevonCmd) -> Gain12/1
  Surface Mixing Function/6(StbdInbdElevonCmd) -> Gain13/1
  Surface Mixing Function/7(PrtOutElevonCmd) -> Gain14/1
  Surface Mixing Function/8(StbdOutdElevonCmd) -> Gain15/1
  Surface Mixing Function/9(ElevatorUtailCmd) -> Gain1/1
  Surface Mixing Function/10(AftFlapCmd) -> Gain2/1
  Surface Mixing Function/11(PylonRudderCmd) -> Gain3/1
  Surface Mixing Function/12(WingletRudderCmd) -> Gain4/1
  Surface Mixing Function/13(UTailRudderCmd) -> Gain5/1
  Surface Mixing Function/4(StbdAileronLowerCmd) -> Gain11/1
  Surface Mixing Function/3(StbdAileronUpperCmd) -> Gain10/1
  Surface Mixing Function/2(PrtAileronLowerCmd) -> Gain9/1
  Surface Mixing Function/1(PrtAileronUpperCmd) -> Gain8/1
  HStab/1 -> Stabilizer_Deg/1, Bus Creator/11  "Sim_StabilizerCmd"
  nmodeTlaLhCmdDeg3/1 -> Spoilers_Deg/1, Bus Creator/10  "Sim_SpoilersCmd"
  SlatLhPosnDeg/1 -> Slats_Deg/1, Bus Creator/9  "Sim_SlatsCmd"
  Gain17/1 -> Bus Creator4/2  "StbdThrottleCmd_Pct"
  Bus Creator4/1 -> "Throttle_Pct "/1
  Gain16/1 -> Bus Creator4/1  "PrtThrottleCmd_Pct"
  Gain15/1 -> Bus Creator3/2  "StbdOutElevonCmd_Deg"
  Gain14/1 -> Bus Creator3/1  "PrtOutElevonCmd_Deg"
  Gain13/1 -> Bus Creator2/2  "StbdInbElevonCmd_Deg"
  Gain12/1 -> Bus Creator2/1  "PrtInbElevonCmd_Deg"
  Gain11/1 -> Bus Creator1/4  "StbdAileronLowerCmd_Deg"
  Gain10/1 -> Bus Creator1/3  "StbdAileronUpperCmd_Deg"
  Gain9/1 -> Bus Creator1/2  "PrtAileronLowerCmd_Deg"
  Gain8/1 -> Bus Creator1/1  "PrtAileronUpperCmd_Deg"
  Bus Creator3/1 -> OutboardElevon_Deg/1
  Bus Creator2/1 -> "InboardElevon_Deg "/1
  Bus Creator1/1 -> "Aileron_Deg "/1
  Variant Model/1(ThrottleCmdOut) -> Gain16/1, Gain17/1  "Sim_ThrottleCmd"
  Throttle/1 -> Variant Model/1(Sim_ThrottleCmd), Bus Creator/4  "Sim_ThrottleCmd"
  Bus Creator/1 -> [Sim_Surface]
  Brake/1 -> Bus Creator/6, Brake (0-1)/1  "Sim_BrakeCmd"
  Nosegear/1 -> Nosegear_Deg/1, Bus Creator/5  "Sim_NosegearCmd"
  Rudder/1 -> Signal Specification2/1, Bus Creator/3  "Sim_RudderCmd"
  Aileron/1 -> Signal Specification/1, Bus Creator/1  "Sim_AileronCmd"
  Elevator/1 -> Signal Specification1/1, Bus Creator/2  "Sim_ElevatorCmd"
  Flap/1 -> Flaps_Deg/1, Bus Creator/7  "Sim_FlapCmd"
  Signal Specification3/1 -> Surface Mixing Function/4(SplitAilCmd)
  Constant2/1 -> Surface Mixing Function/5(elevonBias)
  Constant3/1 -> Surface Mixing Function/6(AileronMax)
